simulink model "test"  (R2021a)
settings: Solver=VariableStepAuto  StartTime=0.0  StopTime=20  MaxStep=1e-4  RelTol=1e-3
values from neighbouring files (symbols this model uses):
  alpha = [0.09877, -0.309, -0.891, 0.5878, 0.7071, -0.8091]    [test_beam_model.m]
  w = [1, 4, 9, 16, 25, 36]    [test_beam_model.m]
  xi = 0.05    [test_beam_model.m]
settings Model: Creator=Alessandro  LastModifiedBy=Alessandro

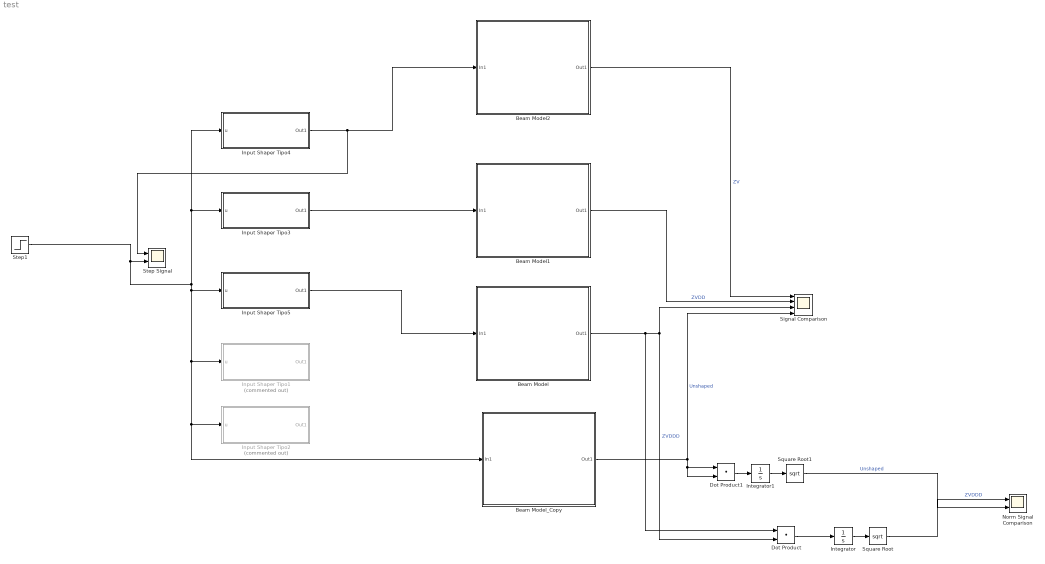
== system test ==
  Beam Model : Subsystem
  Beam Model1 : Subsystem
  Beam Model2 : Subsystem
  Beam Model_Copy : Subsystem
  Dot Product : DotProduct  InputSameDT=on  OutDataTypeStr=Inherit: Inherit via internal rule
  Dot Product1 : DotProduct  InputSameDT=on  OutDataTypeStr=Inherit: Inherit via internal rule
  Input Shaper Tipo1 : Subsystem  Commented=on
  Input Shaper Tipo2 : Subsystem  Commented=on
  Input Shaper Tipo3 : Subsystem
  Input Shaper Tipo4 : Subsystem
  Input Shaper Tipo5 : Subsystem
  Integrator : Integrator
  Integrator1 : Integrator
  Norm Signal Comparison : Scope  NumInputPorts=2
  Signal Comparison : Scope  NumInputPorts=4
  Square Root : Sqrt  SaturateOnIntegerOverflow=on
  Square Root1 : Sqrt  SaturateOnIntegerOverflow=on
  Step Signal : Scope  NumInputPorts=2
  Step1 : Step  Time=2  Before=1  After=0  SampleTime=0
  wires:
  Beam Model/1(Out1) -> Dot Product/2, Signal Comparison/3, Dot Product/1  "ZVDDD"
  Dot Product/1 -> Integrator/1
  Integrator/1 -> Square Root/1
  Integrator1/1 -> Square Root1/1
  Beam Model_Copy/1(Out1) -> Dot Product1/2, Dot Product1/1, Signal Comparison/4  "Unshaped"
  Square Root/1 -> Norm Signal Comparison/1  "ZVDDD"
  Dot Product1/1 -> Integrator1/1
  Square Root1/1 -> Norm Signal Comparison/2  "Unshaped"
  Step1/1 -> Input Shaper Tipo1/1(u), Input Shaper Tipo2/1(u), Beam Model_Copy/1(In1), Input Shaper Tipo5/1(u), Input Shaper Tipo4/1(u), Input Shaper Tipo3/1(u), Step Signal/2
  Input Shaper Tipo5/1(Out1) -> Beam Model/1(In1)
  Input Shaper Tipo3/1(Out1) -> Beam Model1/1(In1)
  Beam Model1/1(Out1) -> Signal Comparison/2  "ZVDD"
  Input Shaper Tipo4/1(Out1) -> Step Signal/1, Beam Model2/1(In1)
  Beam Model2/1(Out1) -> Signal Comparison/1  "ZV"

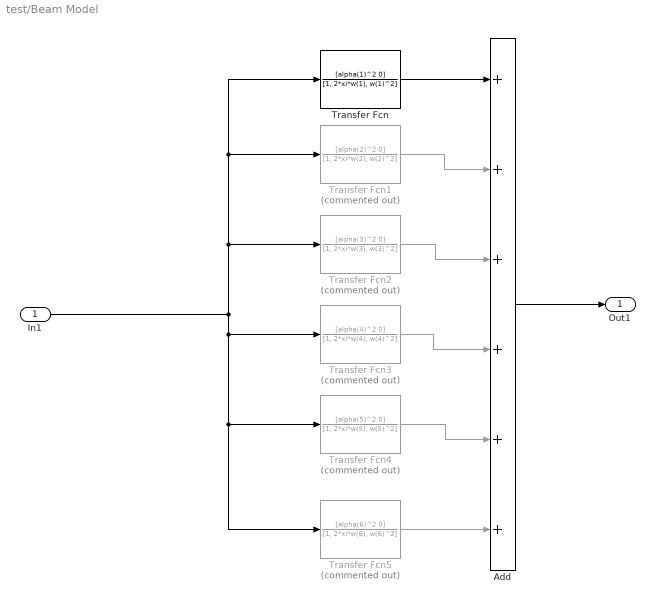
== system test/Beam Model ==
  In1 : Inport
  Add : Sum  Inputs=++++++
  Transfer Fcn : TransferFcn  Numerator=[alpha(1)^2 0]  Denominator=[1, 2*xi*w(1), w(1)^2]
  Transfer Fcn1 : TransferFcn  Commented=on  Numerator=[alpha(2)^2 0]  Denominator=[1, 2*xi*w(2), w(2)^2]
  Transfer Fcn2 : TransferFcn  Commented=on  Numerator=[alpha(3)^2 0]  Denominator=[1, 2*xi*w(3), w(3)^2]
  Transfer Fcn3 : TransferFcn  Commented=on  Numerator=[alpha(4)^2 0]  Denominator=[1, 2*xi*w(4), w(4)^2]
  Transfer Fcn4 : TransferFcn  Commented=on  Numerator=[alpha(5)^2 0]  Denominator=[1, 2*xi*w(5), w(5)^2]
  Transfer Fcn5 : TransferFcn  Commented=on  Numerator=[alpha(6)^2 0]  Denominator=[1, 2*xi*w(6), w(6)^2]
  Out1 : Outport
  wires:
  Transfer Fcn2/1 -> Add/3
  Transfer Fcn4/1 -> Add/5
  Transfer Fcn1/1 -> Add/2
  Add/1 -> Out1/1
  Transfer Fcn/1 -> Add/1
  Transfer Fcn3/1 -> Add/4
  Transfer Fcn5/1 -> Add/6
  In1/1 -> Transfer Fcn5/1, Transfer Fcn4/1, Transfer Fcn3/1, Transfer Fcn/1, Transfer Fcn1/1, Transfer Fcn2/1

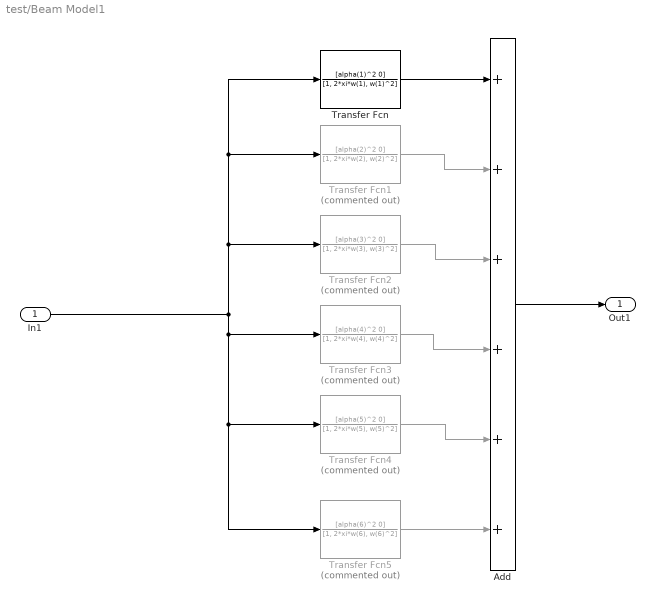
== system test/Beam Model1 ==
  In1 : Inport
  Add : Sum  Inputs=++++++
  Transfer Fcn : TransferFcn  Numerator=[alpha(1)^2 0]  Denominator=[1, 2*xi*w(1), w(1)^2]
  Transfer Fcn1 : TransferFcn  Commented=on  Numerator=[alpha(2)^2 0]  Denominator=[1, 2*xi*w(2), w(2)^2]
  Transfer Fcn2 : TransferFcn  Commented=on  Numerator=[alpha(3)^2 0]  Denominator=[1, 2*xi*w(3), w(3)^2]
  Transfer Fcn3 : TransferFcn  Commented=on  Numerator=[alpha(4)^2 0]  Denominator=[1, 2*xi*w(4), w(4)^2]
  Transfer Fcn4 : TransferFcn  Commented=on  Numerator=[alpha(5)^2 0]  Denominator=[1, 2*xi*w(5), w(5)^2]
  Transfer Fcn5 : TransferFcn  Commented=on  Numerator=[alpha(6)^2 0]  Denominator=[1, 2*xi*w(6), w(6)^2]
  Out1 : Outport
  wires:
  Transfer Fcn2/1 -> Add/3
  Transfer Fcn4/1 -> Add/5
  Transfer Fcn1/1 -> Add/2
  Add/1 -> Out1/1
  Transfer Fcn/1 -> Add/1
  Transfer Fcn3/1 -> Add/4
  Transfer Fcn5/1 -> Add/6
  In1/1 -> Transfer Fcn5/1, Transfer Fcn4/1, Transfer Fcn3/1, Transfer Fcn/1, Transfer Fcn1/1, Transfer Fcn2/1

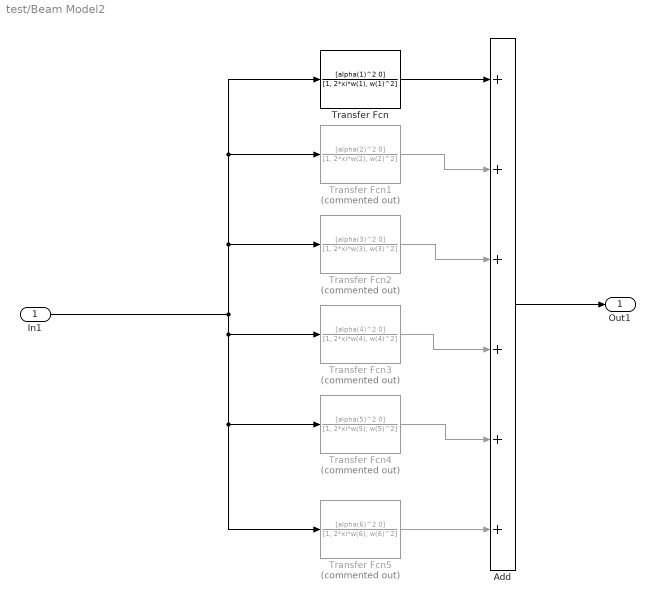
== system test/Beam Model2 ==
  In1 : Inport
  Add : Sum  Inputs=++++++
  Transfer Fcn : TransferFcn  Numerator=[alpha(1)^2 0]  Denominator=[1, 2*xi*w(1), w(1)^2]
  Transfer Fcn1 : TransferFcn  Commented=on  Numerator=[alpha(2)^2 0]  Denominator=[1, 2*xi*w(2), w(2)^2]
  Transfer Fcn2 : TransferFcn  Commented=on  Numerator=[alpha(3)^2 0]  Denominator=[1, 2*xi*w(3), w(3)^2]
  Transfer Fcn3 : TransferFcn  Commented=on  Numerator=[alpha(4)^2 0]  Denominator=[1, 2*xi*w(4), w(4)^2]
  Transfer Fcn4 : TransferFcn  Commented=on  Numerator=[alpha(5)^2 0]  Denominator=[1, 2*xi*w(5), w(5)^2]
  Transfer Fcn5 : TransferFcn  Commented=on  Numerator=[alpha(6)^2 0]  Denominator=[1, 2*xi*w(6), w(6)^2]
  Out1 : Outport
  wires:
  Transfer Fcn2/1 -> Add/3
  Transfer Fcn4/1 -> Add/5
  Transfer Fcn1/1 -> Add/2
  Add/1 -> Out1/1
  Transfer Fcn/1 -> Add/1
  Transfer Fcn3/1 -> Add/4
  Transfer Fcn5/1 -> Add/6
  In1/1 -> Transfer Fcn5/1, Transfer Fcn4/1, Transfer Fcn3/1, Transfer Fcn/1, Transfer Fcn1/1, Transfer Fcn2/1

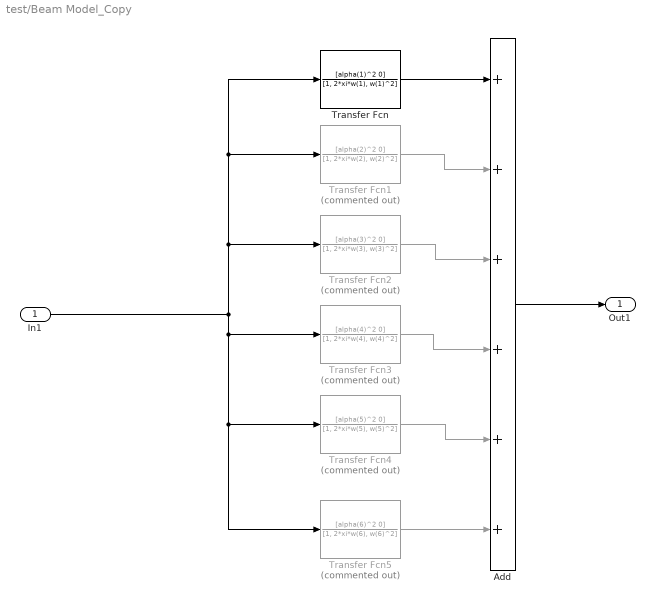
== system test/Beam Model_Copy ==
  In1 : Inport
  Add : Sum  Inputs=++++++
  Transfer Fcn : TransferFcn  Numerator=[alpha(1)^2 0]  Denominator=[1, 2*xi*w(1), w(1)^2]
  Transfer Fcn1 : TransferFcn  Commented=on  Numerator=[alpha(2)^2 0]  Denominator=[1, 2*xi*w(2), w(2)^2]
  Transfer Fcn2 : TransferFcn  Commented=on  Numerator=[alpha(3)^2 0]  Denominator=[1, 2*xi*w(3), w(3)^2]
  Transfer Fcn3 : TransferFcn  Commented=on  Numerator=[alpha(4)^2 0]  Denominator=[1, 2*xi*w(4), w(4)^2]
  Transfer Fcn4 : TransferFcn  Commented=on  Numerator=[alpha(5)^2 0]  Denominator=[1, 2*xi*w(5), w(5)^2]
  Transfer Fcn5 : TransferFcn  Commented=on  Numerator=[alpha(6)^2 0]  Denominator=[1, 2*xi*w(6), w(6)^2]
  Out1 : Outport
  wires:
  Transfer Fcn2/1 -> Add/3
  Transfer Fcn4/1 -> Add/5
  Transfer Fcn1/1 -> Add/2
  Add/1 -> Out1/1
  Transfer Fcn/1 -> Add/1
  Transfer Fcn3/1 -> Add/4
  Transfer Fcn5/1 -> Add/6
  In1/1 -> Transfer Fcn5/1, Transfer Fcn4/1, Transfer Fcn3/1, Transfer Fcn/1, Transfer Fcn1/1, Transfer Fcn2/1

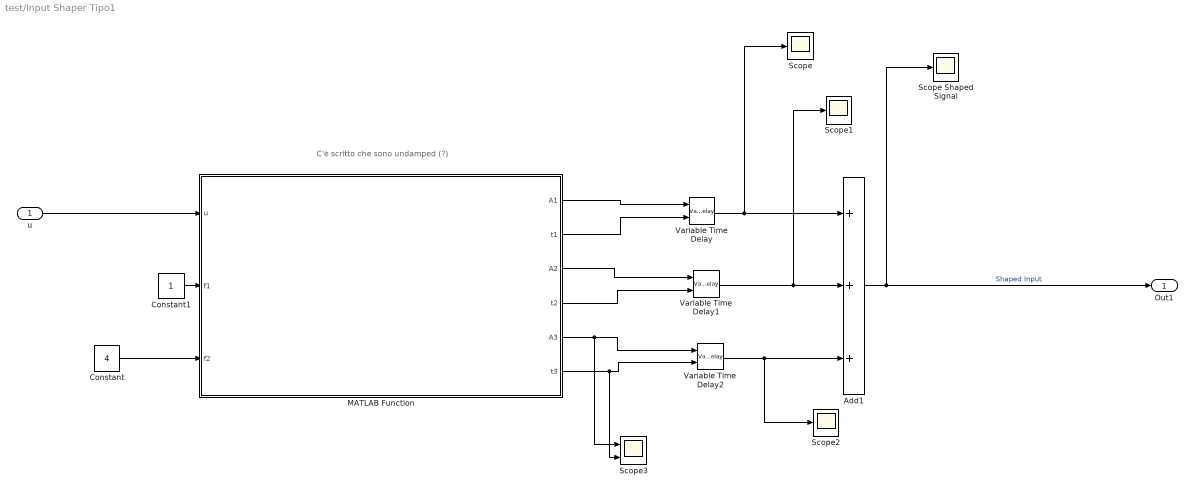
== system test/Input Shaper Tipo1 ==
  note: C'è scritto che sono undamped (?)
  u : Inport
  Add1 : Sum  Inputs=+++
  Constant : Constant  Value=4
  Constant1 : Constant
  MATLAB Function : MATLAB Function  TreatAsAtomicUnit=on
  Scope : Scope
  Scope Shaped Signal : Scope
  Scope1 : Scope
  Scope2 : Scope
  Scope3 : Scope  NumInputPorts=2
  Variable Time Delay : VariableTransportDelay  MaximumDelay=50000  ZeroDelay=on
  Variable Time Delay1 : VariableTransportDelay  MaximumDelay=50000  ZeroDelay=on
  Variable Time Delay2 : VariableTransportDelay  MaximumDelay=50000  ZeroDelay=on
  Out1 : Outport
  wires:
  Constant1/1 -> MATLAB Function/2(f1)
  Variable Time Delay2/1 -> Scope2/1, Add1/3
  MATLAB Function/3(A2) -> Variable Time Delay1/1
  Variable Time Delay1/1 -> Scope1/1, Add1/2
  MATLAB Function/5(A3) -> Scope3/1, Variable Time Delay2/1
  MATLAB Function/4(t2) -> Variable Time Delay1/2
  Constant/1 -> MATLAB Function/3(f2)
  Add1/1 -> Out1/1, Scope Shaped Signal/1  "Shaped Input"
  MATLAB Function/2(t1) -> Variable Time Delay/2
  MATLAB Function/6(t3) -> Scope3/2, Variable Time Delay2/2
  u/1 -> MATLAB Function/1(u)
  Variable Time Delay/1 -> Scope/1, Add1/1
  MATLAB Function/1(A1) -> Variable Time Delay/1

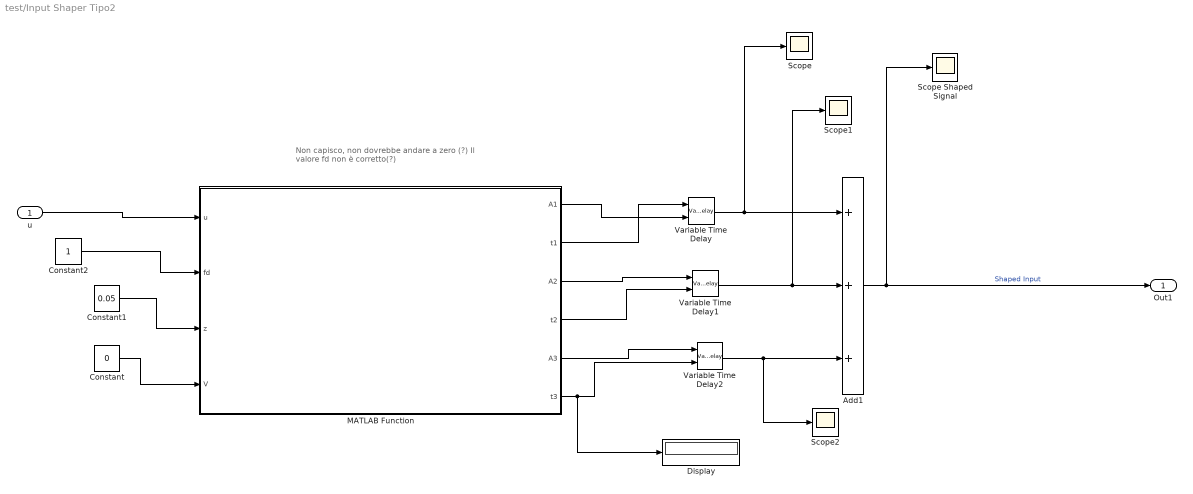
== system test/Input Shaper Tipo2 ==
  note: Non capisco, non dovrebbe andare a zero (?)
      | Il valore fd non è corretto(?)
  u : Inport
  Add1 : Sum  Inputs=+++
  Constant : Constant  Value=0
  Constant1 : Constant  Value=0.05
  Constant2 : Constant
  Display : Display
  MATLAB Function : MATLAB Function  TreatAsAtomicUnit=on
  Scope : Scope
  Scope Shaped Signal : Scope
  Scope1 : Scope
  Scope2 : Scope
  Variable Time Delay : VariableTransportDelay  MaximumDelay=50000  ZeroDelay=on
  Variable Time Delay1 : VariableTransportDelay  MaximumDelay=50000  ZeroDelay=on
  Variable Time Delay2 : VariableTransportDelay  MaximumDelay=50000  ZeroDelay=on
  Out1 : Outport
  wires:
  Constant1/1 -> MATLAB Function/3(z)
  Variable Time Delay2/1 -> Scope2/1, Add1/3
  Variable Time Delay1/1 -> Scope1/1, Add1/2
  Constant/1 -> MATLAB Function/4(V)
  Add1/1 -> Out1/1, Scope Shaped Signal/1  "Shaped Input"
  MATLAB Function/1(A1) -> Variable Time Delay/2
  Variable Time Delay/1 -> Scope/1, Add1/1
  MATLAB Function/2(t1) -> Variable Time Delay/1
  MATLAB Function/3(A2) -> Variable Time Delay1/1
  MATLAB Function/4(t2) -> Variable Time Delay1/2
  MATLAB Function/5(A3) -> Variable Time Delay2/1
  MATLAB Function/6(t3) -> Display/1, Variable Time Delay2/2
  u/1 -> MATLAB Function/1(u)
  Constant2/1 -> MATLAB Function/2(fd)

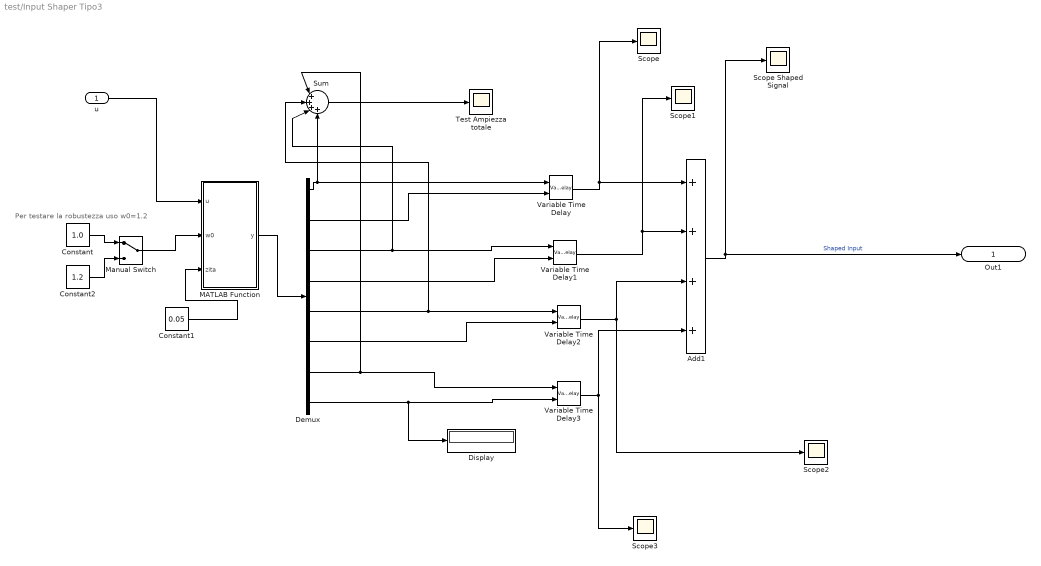
== system test/Input Shaper Tipo3 ==
  note: Per testare la robustezza uso w0=1.2
  u : Inport
  Add1 : Sum  Inputs=++++
  Constant : Constant  Value=1.0
  Constant1 : Constant  Value=0.05
  Constant2 : Constant  Value=1.2
  Demux : Demux  Outputs=8
  Display : Display
  MATLAB Function : MATLAB Function  TreatAsAtomicUnit=on
  Manual Switch : ManualSwitch
  Scope{,1..3} (4 alike) : Scope
  Scope Shaped Signal : Scope
  Sum : Sum  Inputs=|++++
  Test Ampiezza totale : Scope
  Variable Time Delay{,1..3} (4 alike) : VariableTransportDelay  MaximumDelay=50000  ZeroDelay=on
  Out1 : Outport
  wires:
  Variable Time Delay2/1 -> Scope2/1, Add1/3
  Variable Time Delay1/1 -> Scope1/1, Add1/2
  Add1/1 -> Out1/1, Scope Shaped Signal/1  "Shaped Input"
  Demux/2 -> Variable Time Delay/2
  Variable Time Delay/1 -> Scope/1, Add1/1
  Demux/1 -> Variable Time Delay/1, Sum/4
  Demux/3 -> Sum/3, Variable Time Delay1/1
  Demux/4 -> Variable Time Delay1/2
  Demux/5 -> Sum/2, Variable Time Delay2/1
  Demux/6 -> Variable Time Delay2/2
  u/1 -> MATLAB Function/1(u)
  MATLAB Function/1(y) -> Demux/1
  Demux/8 -> Display/1, Variable Time Delay3/2
  Demux/7 -> Variable Time Delay3/1, Sum/1
  Variable Time Delay3/1 -> Scope3/1, Add1/4
  Constant1/1 -> MATLAB Function/3(zita)
  Sum/1 -> Test Ampiezza totale/1
  Constant2/1 -> Manual Switch/2
  Manual Switch/1 -> MATLAB Function/2(w0)
  Constant/1 -> Manual Switch/1

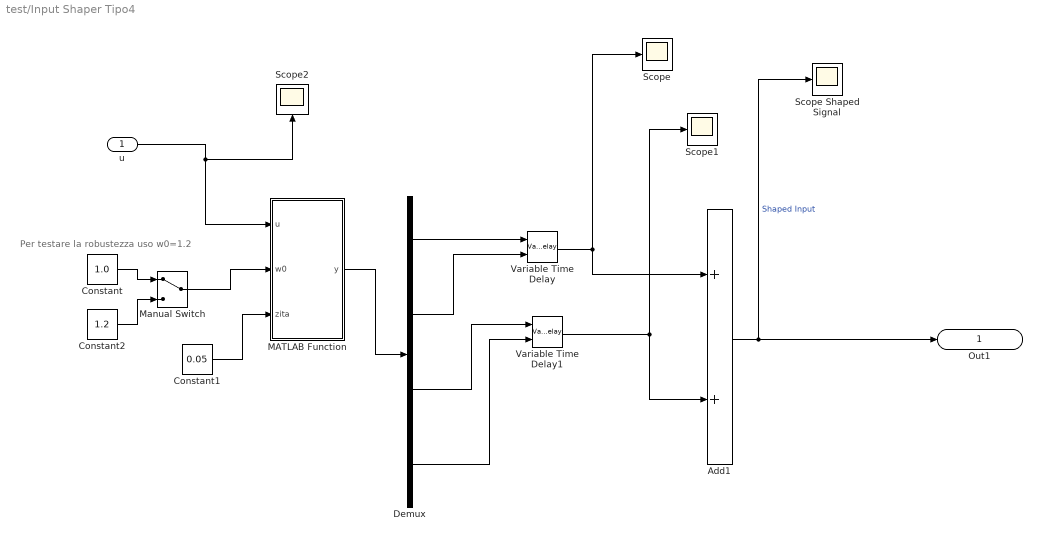
== system test/Input Shaper Tipo4 ==
  note: Per testare la robustezza uso w0=1.2
  u : Inport
  Add1 : Sum
  Constant : Constant  Value=1.0
  Constant1 : Constant  Value=0.05
  Constant2 : Constant  Value=1.2
  Demux : Demux
  MATLAB Function : MATLAB Function  TreatAsAtomicUnit=on
  Manual Switch : ManualSwitch
  Scope : Scope
  Scope Shaped Signal : Scope
  Scope1 : Scope
  Scope2 : Scope
  Variable Time Delay : VariableTransportDelay  MaximumDelay=50000  ZeroDelay=on
  Variable Time Delay1 : VariableTransportDelay  MaximumDelay=50000  ZeroDelay=on
  Out1 : Outport
  wires:
  Variable Time Delay1/1 -> Scope1/1, Add1/2
  Add1/1 -> Scope Shaped Signal/1, Out1/1  "Shaped Input"
  Demux/2 -> Variable Time Delay/2
  Variable Time Delay/1 -> Scope/1, Add1/1
  Demux/1 -> Variable Time Delay/1
  Demux/3 -> Variable Time Delay1/1
  Demux/4 -> Variable Time Delay1/2
  u/1 -> Scope2/1, MATLAB Function/1(u)
  MATLAB Function/1(y) -> Demux/1
  Constant1/1 -> MATLAB Function/3(zita)
  Constant/1 -> Manual Switch/1
  Constant2/1 -> Manual Switch/2
  Manual Switch/1 -> MATLAB Function/2(w0)

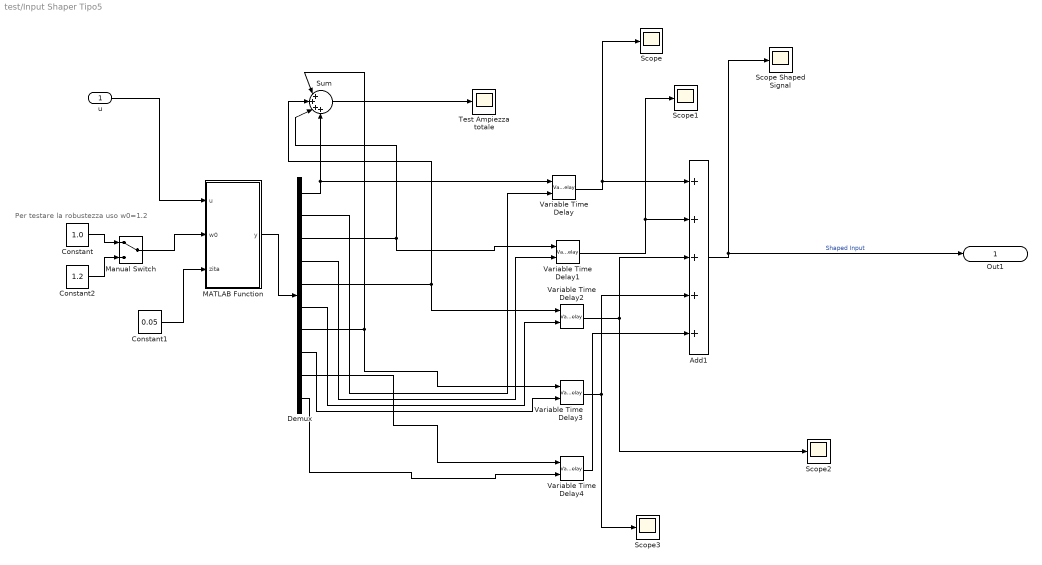
== system test/Input Shaper Tipo5 ==
  note: Per testare la robustezza uso w0=1.2
  u : Inport
  Add1 : Sum  Inputs=+++++
  Constant : Constant  Value=1.0
  Constant1 : Constant  Value=0.05
  Constant2 : Constant  Value=1.2
  Demux : Demux  Outputs=10
  MATLAB Function : MATLAB Function  TreatAsAtomicUnit=on
  Manual Switch : ManualSwitch
  Scope{,1..3} (4 alike) : Scope
  Scope Shaped Signal : Scope
  Sum : Sum  Inputs=|++++
  Test Ampiezza totale : Scope
  Variable Time Delay{,1..4} (5 alike) : VariableTransportDelay  MaximumDelay=50000  ZeroDelay=on
  Out1 : Outport
  wires:
  Variable Time Delay2/1 -> Scope2/1, Add1/3
  Variable Time Delay1/1 -> Scope1/1, Add1/2
  Add1/1 -> Out1/1, Scope Shaped Signal/1  "Shaped Input"
  Demux/2 -> Variable Time Delay/2
  Variable Time Delay/1 -> Scope/1, Add1/1
  Demux/1 -> Variable Time Delay/1, Sum/4
  Demux/3 -> Variable Time Delay1/1, Sum/3
  Demux/4 -> Variable Time Delay1/2
  Demux/5 -> Variable Time Delay2/1, Sum/2
  Demux/6 -> Variable Time Delay2/2
  u/1 -> MATLAB Function/1(u)
  MATLAB Function/1(y) -> Demux/1
  Demux/8 -> Variable Time Delay3/2
  Demux/7 -> Variable Time Delay3/1, Sum/1
  Variable Time Delay3/1 -> Scope3/1, Add1/4
  Constant1/1 -> MATLAB Function/3(zita)
  Sum/1 -> Test Ampiezza totale/1
  Demux/9 -> Variable Time Delay4/1
  Demux/10 -> Variable Time Delay4/2
  Variable Time Delay4/1 -> Add1/5
  Constant2/1 -> Manual Switch/2
  Manual Switch/1 -> MATLAB Function/2(w0)
  Constant/1 -> Manual Switch/1

== matlab function test/Input Shaper Tipo2/MATLAB Function ==
  data: u input; A1 output; fd input; t1 output; A2 output; z input; V input; t2 output; A3 output; t3 output
function [A1,t1,A2,t2,A3,t3] = EI(u,fd,z,V)

% EI(fd,z,V,deltaT) -- Bill Singhose
% Generates an EI shaper for 1 mode.
% The solution comes from a surface fit to data calculated with GAMS.
% The shaper works well over the ranges of 0<V<.2 ans 0<z<.25
% fd - damped frequency (Hz) of vibration being controlled.
% z - damping ratio of vibration being controlled.
% V - vibration limit, for 5% vibration, Vlim=0.05.
% deltaT - time spacing at which input to system is updated.


A1= 0.249684+0.249623*V+0.800081*z+1.23328*V*z+0.495987*z^2+3.17316*V*z^2;
A3 = 0.251489+0.21474*V-0.832493*z+1.41498*V*z+0.851806*z^2-4.90094*V*z^2;
A2 = 1 - (A1+A3);
t1  = 0;
t2  =(0.499899+0.461586*V*z+4.26169*V*z^2+1.75601*V*z^3+8.57843*V^2*z - 108.644*V^2*z^2+336.989*V^2*z^3)/fd;
t3 = 1/fd;
A1=A1*u;
A2=A2*u;
A3=A3*u;
end

== matlab function test/Input Shaper Tipo1/MATLAB Function ==
  data: u input; A1 output; t1 output; A2 output; t2 output; A3 output; t3 output; f1 input; f2 input
function [A1,t1,A2,t2,A3,t3] = InputShaper(u,f1,f2)
% Solves for a 2-mode ZV shaper assuming zero damping in both modes.
%   The result is a 3 impulse sequence.
%   Note that this is NOT the 4 impulse sequence produced by convolving two 
%   ZV shapers together.  
%
%   f1=First Frequency in Hertz
%   f2=Second Frequency in Hertz
%   exactshaper=input shaper sequence [time1 Amp1;time2 Amp2;time3 Amp3]

fL=min([f1 f2]);
fh=max([f1 f2]);
fm=(f1+f2)/2;

% convert to radians/sec
wL=2*pi*fL;wh=2*pi*fh;wm=2*pi*fm;

alpha=cos(pi*(wm-wL)/wm);
A1=1/2/(1+alpha);
A3=A1;
A2=1-2*A1;

A1=A1*u;
A2=A2*u;
A3=A3*u;

T=2*pi/wm;
t1=0;
t2=T/2;
t3=T;

temp=[A1*u,t1; A2*u,t2; A3*u,t3];
end

== matlab function test/Input Shaper Tipo3/MATLAB Function ==
  data: u input; y output; w0 input; zita input
function y = ZVDD_mio(u,w0,zita)
% 1 [Hz] = 2*pi [rad/s] <--- tau_d espressa in s!
% I take w0 as rad/s and convert it.

K=exp((-zita*pi)/sqrt(1-zita^2));
tau_d=2*pi/w0;

A1 = 1/(1+3*K+3*K^2+K^3);
t1 = 0;

A2 = (3*K)/(1+3*K+3*K^2+K^3);
t2 = tau_d/2;

A3 = (3*K^2)/(1+3*K+3*K^2+K^3);
t3 = tau_d;

A4 = K^3/(1+3*K+3*K^2+K^3);
t4 = tau_d*3/2;

A1=u*A1;
A2=u*A2;
A3=u*A3;
A4=u*A4;


y = [A1,t1,A2,t2,A3,t3,A4,t4];

== matlab function test/Input Shaper Tipo4/MATLAB Function ==
  data: u input; y output; w0 input; zita input
function y = ZV_mio(u,w0,zita)
% 1 [Hz] = 2*pi [rad/s] <--- tau_d espressa in s!
% I take w0 as rad/s and convert it.

K=exp((-zita*pi)/sqrt(1-zita^2));
tau_d=2*pi/w0;

A1 = 1/(1+K);
t1 = 0;

A2 = K/(1+K);
t2 = tau_d/2;

A1=u*A1;
A2=u*A2;


y = [A1,t1,A2,t2];

== matlab function test/Input Shaper Tipo5/MATLAB Function ==
  data: u input; y output; w0 input; zita input
function y = ZVDDD_mio(u,w0,zita)
% 1 [Hz] = 2*pi [rad/s] <--- tau_d espressa in s!
% I take w0 as rad/s and convert it.

K=exp((-zita*pi)/sqrt(1-zita^2));
D=1+4*K+6*K^2+4*K^3+K^4;
tau_d=2*pi/w0;

A1 = 1/D;
t1 = 0;

A2 = (4*K)/D;
t2 = tau_d/2;

A3 = (6*K^2)/D;
t3 = tau_d;

A4 = (4*K^3)/D;
t4 = tau_d*3/2;

A5 = K^4/D;
t5 = tau_d*2;

A1=u*A1;
A2=u*A2;
A3=u*A3;
A4=u*A4;
A5=u*A5;


y = [A1,t1,A2,t2,A3,t3,A4,t4,A5,t5];
